simulink model "Filter2017a"  (R2017a)
settings: Solver=VariableStepAuto  StartTime=0.0  StopTime=10  RelTol=1e-3
values from neighbouring files (symbols this model uses):
  Fs = 44100    [Harjoitustyo.m]
  Hr_band = zeros(size(k))    [Harjoitustyo.m]
  Hr_high = ones(size(k))    [Harjoitustyo.m]
  Hr_low = zeros(size(k))    [Harjoitustyo.m]
  M = 64    [BuildFilter_a.m]    (also in Harjoitustyo.m; LuentoEsimerkki.m = 32)
libraries: dspsrcs4 x2
settings Model: Creator=j8889  LastModifiedBy=j8889

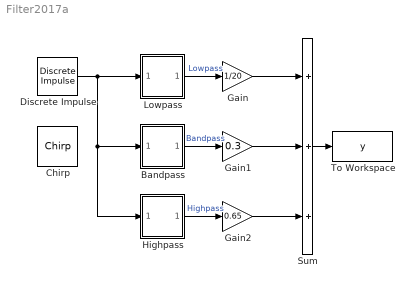
== system Filter2017a ==
  Bandpass : Subsystem
  Chirp : dspsrcs4/Chirp  sweep=Linear  mode=Unidirectional  f0=10  f1=20000  t1=10  Tsweep=50  phase=0  Ts=1/Fs  spf=1  datatype=Double  OutputFrames=off
      settings: SourceProductName=DSP System Toolbox
  Discrete Impulse : dspsrcs4/Discrete  Impulse  Delay=0  SampleTime=1  FrameSample=1  OutputFrames=off  dataType=double  isSigned=on  wordLen=16  udDataType=sfix(16)  fracBitsMode=Best precision  numFracBits=15  OutDataTypeStr=double  LastOutDataTypeStr=double
  Gain : Gain  Gain=1/20
  Gain1 : Gain  Gain=0.3
  Gain2 : Gain  Gain=0.65
  Highpass : Subsystem
  Lowpass : Subsystem
  Sum : Sum  Inputs=+++
  To Workspace : ToWorkspace  VariableName=y  SaveFormat=Timeseries  SampleTime=-1
  wires:
  Sum/1 -> To Workspace/1
  Lowpass/1(Out1) -> Gain/1  "Lowpass"
  Bandpass/1(Out1) -> Gain1/1  "Bandpass"
  Highpass/1(Out1) -> Gain2/1  "Highpass"
  Gain/1 -> Sum/1
  Gain1/1 -> Sum/2
  Gain2/1 -> Sum/3
  Discrete Impulse/1 -> Lowpass/1(In1), Highpass/1(In1), Bandpass/1(In1)

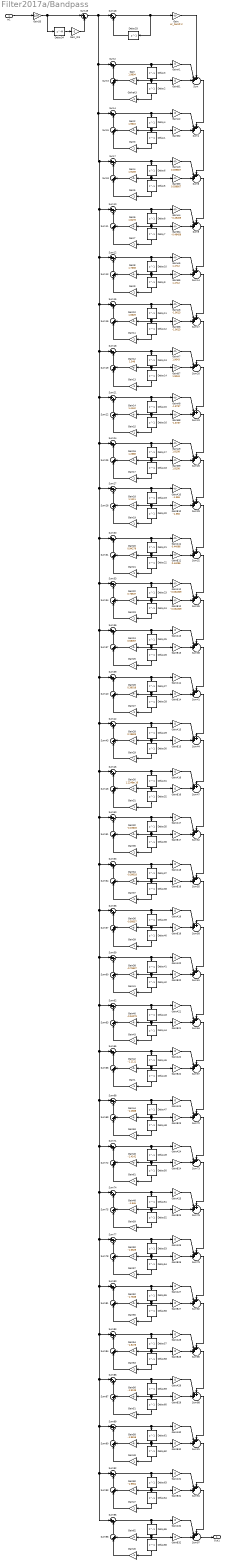
== system Filter2017a/Bandpass ==
  In1 : Inport
  Delay{1..33,35..66} (65 alike) : Delay  DelayLength=1
  Delay34 : Delay  DelayLength=M
  Gaikek3 : Gain  Gain=-1
  Gain : Gain  Gain=1.9904
  Gain{1,3,5,7,9,11,13,15,17,19,21,23,25,27,29,31,35,37,39,41,43,45,47,49,51,53,55,57,59,61,63} (31 alike) : Gain  Gain=-1
  Gain10 : Gain  Gain=1.6629
  Gain12 : Gain  Gain=1.546
  Gain14 : Gain  Gain=1.4142
  Gain16 : Gain  Gain=1.2688
  Gain18 : Gain  Gain=1.1111
  Gain2 : Gain  Gain=1.9616
  Gain20 : Gain  Gain=0.94279
  Gain22 : Gain  Gain=0.76537
  Gain24 : Gain  Gain=0.58057
  Gain26 : Gain  Gain=0.39018
  Gain28 : Gain  Gain=0.19603
  Gain30 : Gain  Gain=1.2246e-16
  Gain32 : Gain  Gain=-0.19603
  Gain33 : Gain  Gain=1/M
  Gain34 : Gain  Gain=-0.39018
  Gain36 : Gain  Gain=-0.58057
  Gain38 : Gain  Gain=-0.76537
  Gain4 : Gain  Gain=1.9139
  Gain40 : Gain  Gain=-0.94279
  Gain42 : Gain  Gain=-1.1111
  Gain44 : Gain  Gain=-1.2688
  Gain46 : Gain  Gain=-1.4142
  Gain48 : Gain  Gain=-1.546
  Gain50 : Gain  Gain=-1.6629
  Gain52 : Gain  Gain=-1.7638
  Gain54 : Gain  Gain=-1.8478
  Gain56 : Gain  Gain=-1.9139
  Gain58 : Gain  Gain=-1.9616
  Gain6 : Gain  Gain=1.8478
  Gain60 : Gain  Gain=-1.9904
  Gain62 : Gain  Gain=-2
  Gain8 : Gain  Gain=1.7638
  GainA{1..2,13..32} (22 alike) : Gain  Gain=0
  GainA10 : Gain  Gain=-1.356
  GainA11 : Gain  Gain=0.44096
  GainA12 : Gain  Gain=-0.034309
  GainA3 : Gain  Gain=0.039807
  GainA4 : Gain  Gain=-0.49459
  GainA5 : Gain  Gain=1.4712
  GainA6 : Gain  Gain=-1.9013
  GainA7 : Gain  Gain=1.9043
  GainA8 : Gain  Gain=-1.8737
  GainA9 : Gain  Gain=1.8108
  GainB{1..2,13..32} (22 alike) : Gain  Gain=0
  GainB10 : Gain  Gain=-1.356
  GainB11 : Gain  Gain=0.44096
  GainB12 : Gain  Gain=-0.034309
  GainB3 : Gain  Gain=0.039807
  GainB4 : Gain  Gain=-0.49459
  GainB5 : Gain  Gain=1.4712
  GainB6 : Gain  Gain=-1.9013
  GainB7 : Gain  Gain=1.9043
  GainB8 : Gain  Gain=-1.8737
  GainB9 : Gain  Gain=1.8108
  Gain_ : Gain  Gain=Hr_band(1)
  Gain_OG : Gain  Gain=-1
  Sum{,1,6,9,14,17,20,23,26,29,32,35,38,41,44,47,52,55,58,61,64,67,70,73,76,79,82,85,88,91,94,97} (32 alike) : Sum  Inputs=+++||
  Sum{2..5,7..8,10..13,15..16,18..19,21..22,24..25,27..28,30..31,33..34,36..37,39..40,42..43,45..46,48..51,53..54,56..57,59..60,62..63,65..66,68..69,71..72,74..75,77..78,80..81,83..84,86..87,89..90,92..93,95..96} (66 alike) : Sum  Inputs=|++
  Out1 : Outport
  wires:
  Sum47/1 -> Sum52/1
  Gain37/1 -> Sum54/1
  Gain34/1 -> Sum54/2
  Sum63/1 -> Sum62/2
  Sum58/1 -> Sum61/1
  GainA21/1 -> Sum64/2
  Delay38/1 -> Gain37/1
  Gain43/1 -> Sum63/1
  Sum54/1 -> Sum53/2
  Delay37/1 -> Delay38/1, Gain34/1, GainB18/1
  GainA18/1 -> Sum55/2
  GainB21/1 -> Sum64/3
  Sum52/1 -> Sum55/1
  Delay50/1 -> Gain61/1
  Gain32/1 -> Sum51/2
  Delay64/1 -> Gain47/1
  Delay54/1 -> Gain57/1
  Delay52/1 -> Gain59/1
  GainA19/1 -> Sum58/2
  Gain_OG/1 -> Sum49/2
  Delay62/1 -> Gain49/1
  Delay58/1 -> Gain53/1
  Sum76/1 -> Sum79/1
  Gain54/1 -> Sum84/2
  GainB24/1 -> Sum73/3
  Sum75/1 -> Sum74/2
  Sum78/1 -> Sum77/2
  Sum72/1 -> Sum71/2
  Sum80/1 -> Delay55/1, GainA27/1
  Gain57/1 -> Sum78/1
  GainA27/1 -> Sum82/2
  Gain52/1 -> Sum81/2
  Sum91/1 -> Sum94/1
  Delay55/1 -> Delay56/1, Gain52/1, GainB27/1
  Sum84/1 -> Sum83/2
  Sum93/1 -> Sum92/2
  Sum71/1 -> GainA24/1, Delay49/1
  Sum66/1 -> Sum65/2
  GainB28/1 -> Sum85/3
  Sum69/1 -> Sum68/2
  Sum92/1 -> Delay63/1, GainA31/1
  GainB25/1 -> Sum76/3
  Delay47/1 -> Delay48/1, Gain44/1, GainB23/1
  Gain49/1 -> Sum90/1
  GainA28/1 -> Sum85/2
  Sum77/1 -> GainA26/1, Delay53/1
  Delay61/1 -> GainB30/1, Gain58/1, Delay62/1
  Gain58/1 -> Sum90/2
  Delay45/1 -> GainB22/1, Gain42/1, Delay46/1
  Sum83/1 -> GainA28/1, Delay57/1
  GainA24/1 -> Sum73/2
  Gain42/1 -> Sum66/2
  Gain48/1 -> Sum75/2
  Delay66/1 -> Gain45/1
  Sum97/1 -> Out1/1
  Delay60/1 -> Gain51/1
  GainB17/1 -> Sum52/3
  Sum70/1 -> Sum73/1
  Gain39/1 -> Sum57/1
  Gain60/1 -> Sum93/2
  Sum59/1 -> Delay41/1, GainA20/1
  Delay41/1 -> Delay42/1, Gain38/1, GainB20/1
  Gain38/1 -> Sum60/2
  GainB26/1 -> Sum79/3
  Delay36/1 -> Gain35/1
  Gain35/1 -> Sum51/1
  Sum50/1 -> GainA17/1, Delay35/1
  Sum60/1 -> Sum59/2
  Sum65/1 -> GainA22/1, Delay45/1
  GainA22/1 -> Sum67/2
  GainA20/1 -> Sum61/2
  Gain41/1 -> Sum60/1
  Sum81/1 -> Sum80/2
  Sum55/1 -> Sum58/1
  Sum68/1 -> Delay47/1, GainA23/1
  Sum57/1 -> Sum56/2
  Gain36/1 -> Sum57/2
  Delay42/1 -> Gain41/1
  Gain1/1 -> Sum66/1
  GainB31/1 -> Sum94/3
  Sum64/1 -> Sum67/1
  GainB16/1 -> Sum47/3
  Delay63/1 -> Delay64/1, Gain60/1, GainB31/1
  Gain30/1 -> Sum46/2
  Sum/1 -> Sum1/1
  GainA31/1 -> Sum94/2
  Gain18/1 -> Sum28/2
  Gain25/1 -> Sum37/1
  Sum35/1 -> Sum38/1
  Sum94/1 -> Sum97/1
  Gain23/1 -> Sum34/1
  Delay32/1 -> Gain31/1
  Sum25/1 -> Sum24/2
  Gain44/1 -> Sum69/2
  Gain27/1 -> Sum40/1
  Delay13/1 -> GainB7/1, Gain12/1, Delay14/1
  GainB23/1 -> Sum70/3
  GainB5/1 -> Sum14/3
  GainA2/1 -> Sum1/2
  Gain6/1 -> Sum11/2
  Gain13/1 -> Sum19/1
  Delay27/1 -> Delay28/1, Gain26/1, GainB14/1
  Sum16/1 -> Sum15/2
  Gain55/1 -> Sum81/1
  Delay19/1 -> Delay20/1, Gain18/1, GainB10/1
  Delay25/1 -> GainB13/1, Gain24/1, Delay26/1
  Delay39/1 -> GainB19/1, Gain36/1, Delay40/1
  GainB7/1 -> Sum20/3
  Sum46/1 -> Sum45/2
  Delay16/1 -> Gain15/1
  GainA9/1 -> Sum26/2
  Sum36/1 -> GainA13/1, Delay25/1
  Sum73/1 -> Sum76/1
  Delay7/1 -> Gain7/1
  Sum6/1 -> Sum9/1
  Gain7/1 -> Sum11/1
  Delay29/1 -> GainB15/1, Gain28/1, Delay30/1
  Sum49/1 -> Sum4/1, Sum50/1, Sum53/1, Sum56/1, Sum59/1, Sum68/1, Sum71/1, Sum74/1, Sum77/1, Sum80/1, Sum83/1, Sum95/1, Sum92/1, Sum89/1, Sum86/1, Sum65/1, Sum62/1, Sum45/1, Sum42/1, Sum39/1, Sum36/1, Sum33/1, Sum30/1, Sum27/1, Sum24/1, Sum21/1, Sum18/1, Sum15/1, Sum12/1, Sum10/1, Sum7/1, Sum2/1, Sum48/1
  GainA3/1 -> Sum6/2
  Sum7/1 -> GainA3/1, Delay6/1
  Delay3/1 -> GainB1/1, Gain/1, Delay2/1
  GainB22/1 -> Sum67/3
  Delay1/1 -> Gain3/1
  GainB3/1 -> Sum6/3
  Sum33/1 -> Delay23/1, GainA12/1
  Gaikek3/1 -> Sum3/1
  Sum3/1 -> Sum2/2
  Sum11/1 -> Sum10/2
  Gain12/1 -> Sum19/2
  Gain26/1 -> Sum40/2
  Delay35/1 -> GainB17/1, Gain32/1, Delay36/1
  Sum48/1 -> Gain_/1, Delay33/1
  Gain22/1 -> Sum34/2
  Gain10/1 -> Sum16/2
  Sum43/1 -> Sum42/2
  Delay57/1 -> GainB28/1, Gain54/1, Delay58/1
  Delay6/1 -> GainB3/1, Gain4/1, Delay5/1
  Delay2/1 -> Gaikek3/1
  Delay51/1 -> Delay52/1, Gain48/1, GainB25/1
  Gain11/1 -> Sum16/1
  GainB27/1 -> Sum82/3
  Sum4/1 -> Delay4/1, GainA2/1
  Gain47/1 -> Sum93/1
  Sum53/1 -> Delay37/1, GainA18/1
  Sum13/1 -> Sum12/2
  Gain50/1 -> Sum78/2
  GainA1/1 -> Sum/2
  Gain51/1 -> Sum87/1
  GainB30/1 -> Sum91/3
  Gain31/1 -> Sum46/1
  Delay22/1 -> Gain21/1
  Gain20/1 -> Sum31/2
  Gain63/1 -> Sum69/1
  GainB13/1 -> Sum38/3
  GainA26/1 -> Sum79/2
  GainB20/1 -> Sum61/3
  Sum10/1 -> Delay8/1, GainA4/1
  Gain45/1 -> Sum96/1
  Delay30/1 -> Gain29/1
  Sum34/1 -> Sum33/2
  Sum88/1 -> Sum91/1
  Delay48/1 -> Gain63/1
  Sum19/1 -> Sum18/2
  Gain5/1 -> Sum8/1
  GainB18/1 -> Sum55/3
  Delay40/1 -> Gain39/1
  Sum90/1 -> Sum89/2
  Sum89/1 -> GainA30/1, Delay61/1
  Gain19/1 -> Sum28/1
  GainA6/1 -> Sum17/2
  Sum20/1 -> Sum23/1
  Sum39/1 -> Delay27/1, GainA14/1
  GainB14/1 -> Sum41/3
  GainA25/1 -> Sum76/2
  Sum74/1 -> Delay51/1, GainA25/1
  Sum18/1 -> GainA7/1, Delay13/1
  GainA8/1 -> Sum23/2
  Sum29/1 -> Sum32/1
  Sum1/1 -> Sum6/1
  Sum5/1 -> Sum4/2
  Delay26/1 -> Gain25/1
  Gain46/1 -> Sum72/2
  Sum12/1 -> GainA5/1, Delay10/1
  Gain61/1 -> Sum72/1
  Gain8/1 -> Sum13/2
  Delay33/1 -> Sum48/2
  Sum38/1 -> Sum41/1
  GainB4/1 -> Sum9/3
  Sum24/1 -> GainA9/1, Delay17/1
  GainA5/1 -> Sum14/2
  Delay14/1 -> Gain13/1
  GainB6/1 -> Sum17/3
  Gain14/1 -> Sum22/2
  Sum22/1 -> Sum21/2
  Delay20/1 -> Gain19/1
  GainB2/1 -> Sum1/3
  Delay8/1 -> Delay7/1, Gain6/1, GainB4/1
  Sum56/1 -> GainA19/1, Delay39/1
  GainA12/1 -> Sum35/2
  Sum82/1 -> Sum85/1
  GainA14/1 -> Sum41/2
  Delay34/1 -> Gain_OG/1
  Delay17/1 -> GainB9/1, Gain16/1, Delay18/1
  Sum23/1 -> Sum26/1
  Gain/1 -> Sum3/2
  GainA30/1 -> Sum91/2
  Delay24/1 -> Gain23/1
  GainA4/1 -> Sum9/2
  GainA16/1 -> Sum47/2
  GainB9/1 -> Sum26/3
  Sum9/1 -> Sum14/1
  Gain17/1 -> Sum25/1
  Delay44/1 -> Gain43/1
  In1/1 -> Gain33/1
  GainA23/1 -> Sum70/2
  Sum21/1 -> Delay15/1, GainA8/1
  Delay28/1 -> Gain27/1
  Gain24/1 -> Sum37/2
  Sum15/1 -> Delay11/1, GainA6/1
  GainB12/1 -> Sum35/3
  GainB10/1 -> Sum29/3
  Sum14/1 -> Sum17/1
  Delay4/1 -> Delay1/1, Gain2/1, GainB2/1
  GainA10/1 -> Sum29/2
  Delay43/1 -> GainB21/1, Gain40/1, Delay44/1
  GainB11/1 -> Sum32/3
  GainA13/1 -> Sum38/2
  GainB15/1 -> Sum44/3
  Gain59/1 -> Sum75/1
  Sum79/1 -> Sum82/1
  Delay10/1 -> GainB5/1, Gain8/1, Delay9/1
  Sum37/1 -> Sum36/2
  Sum40/1 -> Sum39/2
  Delay11/1 -> Delay12/1, Gain10/1, GainB6/1
  Sum30/1 -> GainA11/1, Delay21/1
  Sum17/1 -> Sum20/1
  Delay31/1 -> Delay32/1, Gain30/1, GainB16/1
  Delay15/1 -> Delay16/1, Gain14/1, GainB8/1
  Gain40/1 -> Sum63/2
  Sum42/1 -> GainA15/1, Delay29/1
  Gain2/1 -> Sum5/2
  Sum51/1 -> Sum50/2
  Gain15/1 -> Sum22/1
  Delay56/1 -> Gain55/1
  GainA7/1 -> Sum20/2
  Sum44/1 -> Sum47/1
  Sum8/1 -> Sum7/2
  Delay23/1 -> Delay24/1, Gain22/1, GainB12/1
  Gain16/1 -> Sum25/2
  Sum45/1 -> Delay31/1, GainA16/1
  Delay21/1 -> GainB11/1, Gain20/1, Delay22/1
  GainB1/1 -> Sum/3
  Delay18/1 -> Gain17/1
  Gain29/1 -> Sum43/1
  Gain4/1 -> Sum8/2
  Gain21/1 -> Sum31/1
  Sum27/1 -> Delay19/1, GainA10/1
  Gain28/1 -> Sum43/2
  Sum28/1 -> Sum27/2
  Delay5/1 -> Gain5/1
  Sum61/1 -> Sum64/1
  Gain56/1 -> Sum87/2
  GainB19/1 -> Sum58/3
  Sum85/1 -> Sum88/1
  Gain53/1 -> Sum84/1
  Sum41/1 -> Sum44/1
  Gain9/1 -> Sum13/1
  Delay59/1 -> Delay60/1, Gain56/1, GainB29/1
  GainA11/1 -> Sum32/2
  Sum2/1 -> GainA1/1, Delay3/1
  Sum67/1 -> Sum70/1
  GainB29/1 -> Sum88/3
  Sum87/1 -> Sum86/2
  Gain3/1 -> Sum5/1
  Sum96/1 -> Sum95/2
  Delay53/1 -> GainB26/1, Gain50/1, Delay54/1
  GainA29/1 -> Sum88/2
  GainA15/1 -> Sum44/2
  Sum26/1 -> Sum29/1
  Sum31/1 -> Sum30/2
  Delay12/1 -> Gain11/1
  Sum86/1 -> Delay59/1, GainA29/1
  Delay9/1 -> Gain9/1
  Gain33/1 -> Delay34/1, Sum49/1
  Delay46/1 -> Gain1/1
  GainB32/1 -> Sum97/3
  Sum32/1 -> Sum35/1
  Delay49/1 -> GainB24/1, Gain46/1, Delay50/1
  Sum62/1 -> GainA21/1, Delay43/1
  GainB8/1 -> Sum23/3
  Delay65/1 -> GainB32/1, Gain62/1, Delay66/1
  Gain62/1 -> Sum96/2
  Sum95/1 -> GainA32/1, Delay65/1
  GainA32/1 -> Sum97/2
  GainA17/1 -> Sum52/2
  Gain_/1 -> Sum/1

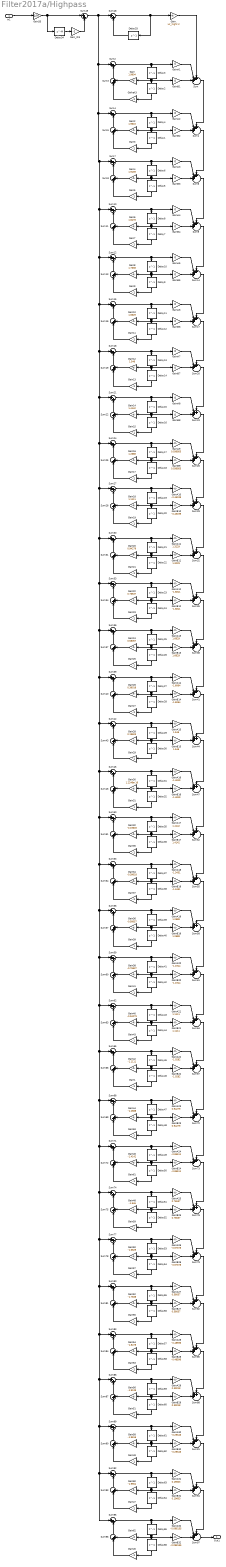
== system Filter2017a/Highpass ==
  In1 : Inport
  Delay{1..33,35..66} (65 alike) : Delay  DelayLength=1
  Delay34 : Delay  DelayLength=M
  Gaikek3 : Gain  Gain=-1
  Gain : Gain  Gain=1.9904
  Gain{1,3,5,7,9,11,13,15,17,19,21,23,25,27,29,31,35,37,39,41,43,45,47,49,51,53,55,57,59,61,63} (31 alike) : Gain  Gain=-1
  Gain10 : Gain  Gain=1.6629
  Gain12 : Gain  Gain=1.546
  Gain14 : Gain  Gain=1.4142
  Gain16 : Gain  Gain=1.2688
  Gain18 : Gain  Gain=1.1111
  Gain2 : Gain  Gain=1.9616
  Gain20 : Gain  Gain=0.94279
  Gain22 : Gain  Gain=0.76537
  Gain24 : Gain  Gain=0.58057
  Gain26 : Gain  Gain=0.39018
  Gain28 : Gain  Gain=0.19603
  Gain30 : Gain  Gain=1.2246e-16
  Gain32 : Gain  Gain=-0.19603
  Gain33 : Gain  Gain=1/M
  Gain34 : Gain  Gain=-0.39018
  Gain36 : Gain  Gain=-0.58057
  Gain38 : Gain  Gain=-0.76537
  Gain4 : Gain  Gain=1.9139
  Gain40 : Gain  Gain=-0.94279
  Gain42 : Gain  Gain=-1.1111
  Gain44 : Gain  Gain=-1.2688
  Gain46 : Gain  Gain=-1.4142
  Gain48 : Gain  Gain=-1.546
  Gain50 : Gain  Gain=-1.6629
  Gain52 : Gain  Gain=-1.7638
  Gain54 : Gain  Gain=-1.8478
  Gain56 : Gain  Gain=-1.9139
  Gain58 : Gain  Gain=-1.9616
  Gain6 : Gain  Gain=1.8478
  Gain60 : Gain  Gain=-1.9904
  Gain62 : Gain  Gain=-2
  Gain8 : Gain  Gain=1.7638
  GainA{1..8} (8 alike) : Gain  Gain=0
  GainA10 : Gain  Gain=-0.45199
  GainA11 : Gain  Gain=1.3229
  GainA12 : Gain  Gain=-1.6811
  GainA13 : Gain  Gain=1.6629
  GainA14 : Gain  Gain=-1.6064
  GainA15 : Gain  Gain=1.546
  GainA16 : Gain  Gain=-1.4819
  GainA17 : Gain  Gain=1.4142
  GainA18 : Gain  Gain=-1.3431
  GainA19 : Gain  Gain=1.2688
  GainA20 : Gain  Gain=-1.1914
  GainA21 : Gain  Gain=1.1111
  GainA22 : Gain  Gain=-1.0282
  GainA23 : Gain  Gain=0.94279
  GainA24 : Gain  Gain=-0.85511
  GainA25 : Gain  Gain=0.76537
  GainA26 : Gain  Gain=-0.67378
  GainA27 : Gain  Gain=0.58057
  GainA28 : Gain  Gain=-0.48596
  GainA29 : Gain  Gain=0.39018
  GainA30 : Gain  Gain=-0.29346
  GainA31 : Gain  Gain=0.19603
  GainA32 : Gain  Gain=-0.098135
  GainA9 : Gain  Gain=0.036955
  GainB{1..8} (8 alike) : Gain  Gain=0
  GainB10 : Gain  Gain=-0.45199
  GainB11 : Gain  Gain=1.3229
  GainB12 : Gain  Gain=-1.6811
  GainB13 : Gain  Gain=1.6629
  GainB14 : Gain  Gain=-1.6064
  GainB15 : Gain  Gain=1.546
  GainB16 : Gain  Gain=-1.4819
  GainB17 : Gain  Gain=1.4142
  GainB18 : Gain  Gain=-1.3431
  GainB19 : Gain  Gain=1.2688
  GainB20 : Gain  Gain=-1.1914
  GainB21 : Gain  Gain=1.1111
  GainB22 : Gain  Gain=-1.0282
  GainB23 : Gain  Gain=0.94279
  GainB24 : Gain  Gain=-0.85511
  GainB25 : Gain  Gain=0.76537
  GainB26 : Gain  Gain=-0.67378
  GainB27 : Gain  Gain=0.58057
  GainB28 : Gain  Gain=-0.48596
  GainB29 : Gain  Gain=0.39018
  GainB30 : Gain  Gain=-0.29346
  GainB31 : Gain  Gain=0.19603
  GainB32 : Gain  Gain=-0.098135
  GainB9 : Gain  Gain=0.036955
  Gain_ : Gain  Gain=Hr_high(1)
  Gain_OG : Gain  Gain=-1
  Sum{,1,6,9,14,17,20,23,26,29,32,35,38,41,44,47,52,55,58,61,64,67,70,73,76,79,82,85,88,91,94,97} (32 alike) : Sum  Inputs=+++||
  Sum{2..5,7..8,10..13,15..16,18..19,21..22,24..25,27..28,30..31,33..34,36..37,39..40,42..43,45..46,48..51,53..54,56..57,59..60,62..63,65..66,68..69,71..72,74..75,77..78,80..81,83..84,86..87,89..90,92..93,95..96} (66 alike) : Sum  Inputs=|++
  Out1 : Outport
  wires:
  Sum47/1 -> Sum52/1
  Gain37/1 -> Sum54/1
  Gain34/1 -> Sum54/2
  Sum63/1 -> Sum62/2
  Sum58/1 -> Sum61/1
  GainA21/1 -> Sum64/2
  Delay38/1 -> Gain37/1
  Gain43/1 -> Sum63/1
  Sum54/1 -> Sum53/2
  Delay37/1 -> Delay38/1, Gain34/1, GainB18/1
  GainA18/1 -> Sum55/2
  GainB21/1 -> Sum64/3
  Sum52/1 -> Sum55/1
  Delay50/1 -> Gain61/1
  Gain32/1 -> Sum51/2
  Delay64/1 -> Gain47/1
  Delay54/1 -> Gain57/1
  Delay52/1 -> Gain59/1
  GainA19/1 -> Sum58/2
  Gain_OG/1 -> Sum49/2
  Delay62/1 -> Gain49/1
  Delay58/1 -> Gain53/1
  Sum76/1 -> Sum79/1
  Gain54/1 -> Sum84/2
  GainB24/1 -> Sum73/3
  Sum75/1 -> Sum74/2
  Sum78/1 -> Sum77/2
  Sum72/1 -> Sum71/2
  Sum80/1 -> Delay55/1, GainA27/1
  Gain57/1 -> Sum78/1
  GainA27/1 -> Sum82/2
  Gain52/1 -> Sum81/2
  Sum91/1 -> Sum94/1
  Delay55/1 -> Delay56/1, Gain52/1, GainB27/1
  Sum84/1 -> Sum83/2
  Sum93/1 -> Sum92/2
  Sum71/1 -> GainA24/1, Delay49/1
  Sum66/1 -> Sum65/2
  GainB28/1 -> Sum85/3
  Sum69/1 -> Sum68/2
  Sum92/1 -> Delay63/1, GainA31/1
  GainB25/1 -> Sum76/3
  Delay47/1 -> Delay48/1, Gain44/1, GainB23/1
  Gain49/1 -> Sum90/1
  GainA28/1 -> Sum85/2
  Sum77/1 -> GainA26/1, Delay53/1
  Delay61/1 -> GainB30/1, Gain58/1, Delay62/1
  Gain58/1 -> Sum90/2
  Delay45/1 -> GainB22/1, Gain42/1, Delay46/1
  Sum83/1 -> GainA28/1, Delay57/1
  GainA24/1 -> Sum73/2
  Gain42/1 -> Sum66/2
  Gain48/1 -> Sum75/2
  Delay66/1 -> Gain45/1
  Sum97/1 -> Out1/1
  Delay60/1 -> Gain51/1
  GainB17/1 -> Sum52/3
  Sum70/1 -> Sum73/1
  Gain39/1 -> Sum57/1
  Gain60/1 -> Sum93/2
  Sum59/1 -> Delay41/1, GainA20/1
  Delay41/1 -> Delay42/1, Gain38/1, GainB20/1
  Gain38/1 -> Sum60/2
  GainB26/1 -> Sum79/3
  Delay36/1 -> Gain35/1
  Gain35/1 -> Sum51/1
  Sum50/1 -> GainA17/1, Delay35/1
  Sum60/1 -> Sum59/2
  Sum65/1 -> GainA22/1, Delay45/1
  GainA22/1 -> Sum67/2
  GainA20/1 -> Sum61/2
  Gain41/1 -> Sum60/1
  Sum81/1 -> Sum80/2
  Sum55/1 -> Sum58/1
  Sum68/1 -> Delay47/1, GainA23/1
  Sum57/1 -> Sum56/2
  Gain36/1 -> Sum57/2
  Delay42/1 -> Gain41/1
  Gain1/1 -> Sum66/1
  GainB31/1 -> Sum94/3
  Sum64/1 -> Sum67/1
  GainB16/1 -> Sum47/3
  Delay63/1 -> Delay64/1, Gain60/1, GainB31/1
  Gain30/1 -> Sum46/2
  Sum/1 -> Sum1/1
  GainA31/1 -> Sum94/2
  Gain18/1 -> Sum28/2
  Gain25/1 -> Sum37/1
  Sum35/1 -> Sum38/1
  Sum94/1 -> Sum97/1
  Gain23/1 -> Sum34/1
  Delay32/1 -> Gain31/1
  Sum25/1 -> Sum24/2
  Gain44/1 -> Sum69/2
  Gain27/1 -> Sum40/1
  Delay13/1 -> GainB7/1, Gain12/1, Delay14/1
  GainB23/1 -> Sum70/3
  GainB5/1 -> Sum14/3
  GainA2/1 -> Sum1/2
  Gain6/1 -> Sum11/2
  Gain13/1 -> Sum19/1
  Delay27/1 -> Delay28/1, Gain26/1, GainB14/1
  Sum16/1 -> Sum15/2
  Gain55/1 -> Sum81/1
  Delay19/1 -> Delay20/1, Gain18/1, GainB10/1
  Delay25/1 -> GainB13/1, Gain24/1, Delay26/1
  Delay39/1 -> GainB19/1, Gain36/1, Delay40/1
  GainB7/1 -> Sum20/3
  Sum46/1 -> Sum45/2
  Delay16/1 -> Gain15/1
  GainA9/1 -> Sum26/2
  Sum36/1 -> GainA13/1, Delay25/1
  Sum73/1 -> Sum76/1
  Delay7/1 -> Gain7/1
  Sum6/1 -> Sum9/1
  Gain7/1 -> Sum11/1
  Delay29/1 -> GainB15/1, Gain28/1, Delay30/1
  Sum49/1 -> Sum4/1, Sum50/1, Sum53/1, Sum56/1, Sum59/1, Sum68/1, Sum71/1, Sum74/1, Sum77/1, Sum80/1, Sum83/1, Sum95/1, Sum92/1, Sum89/1, Sum86/1, Sum65/1, Sum62/1, Sum45/1, Sum42/1, Sum39/1, Sum36/1, Sum33/1, Sum30/1, Sum27/1, Sum24/1, Sum21/1, Sum18/1, Sum15/1, Sum12/1, Sum10/1, Sum7/1, Sum2/1, Sum48/1
  GainA3/1 -> Sum6/2
  Sum7/1 -> GainA3/1, Delay6/1
  Delay3/1 -> GainB1/1, Gain/1, Delay2/1
  GainB22/1 -> Sum67/3
  Delay1/1 -> Gain3/1
  GainB3/1 -> Sum6/3
  Sum33/1 -> Delay23/1, GainA12/1
  Gaikek3/1 -> Sum3/1
  Sum3/1 -> Sum2/2
  Sum11/1 -> Sum10/2
  Gain12/1 -> Sum19/2
  Gain26/1 -> Sum40/2
  Delay35/1 -> GainB17/1, Gain32/1, Delay36/1
  Sum48/1 -> Gain_/1, Delay33/1
  Gain22/1 -> Sum34/2
  Gain10/1 -> Sum16/2
  Sum43/1 -> Sum42/2
  Delay57/1 -> GainB28/1, Gain54/1, Delay58/1
  Delay6/1 -> GainB3/1, Gain4/1, Delay5/1
  Delay2/1 -> Gaikek3/1
  Delay51/1 -> Delay52/1, Gain48/1, GainB25/1
  Gain11/1 -> Sum16/1
  GainB27/1 -> Sum82/3
  Sum4/1 -> Delay4/1, GainA2/1
  Gain47/1 -> Sum93/1
  Sum53/1 -> Delay37/1, GainA18/1
  Sum13/1 -> Sum12/2
  Gain50/1 -> Sum78/2
  GainA1/1 -> Sum/2
  Gain51/1 -> Sum87/1
  GainB30/1 -> Sum91/3
  Gain31/1 -> Sum46/1
  Delay22/1 -> Gain21/1
  Gain20/1 -> Sum31/2
  Gain63/1 -> Sum69/1
  GainB13/1 -> Sum38/3
  GainA26/1 -> Sum79/2
  GainB20/1 -> Sum61/3
  Sum10/1 -> Delay8/1, GainA4/1
  Gain45/1 -> Sum96/1
  Delay30/1 -> Gain29/1
  Sum34/1 -> Sum33/2
  Sum88/1 -> Sum91/1
  Delay48/1 -> Gain63/1
  Sum19/1 -> Sum18/2
  Gain5/1 -> Sum8/1
  GainB18/1 -> Sum55/3
  Delay40/1 -> Gain39/1
  Sum90/1 -> Sum89/2
  Sum89/1 -> GainA30/1, Delay61/1
  Gain19/1 -> Sum28/1
  GainA6/1 -> Sum17/2
  Sum20/1 -> Sum23/1
  Sum39/1 -> Delay27/1, GainA14/1
  GainB14/1 -> Sum41/3
  GainA25/1 -> Sum76/2
  Sum74/1 -> Delay51/1, GainA25/1
  Sum18/1 -> GainA7/1, Delay13/1
  GainA8/1 -> Sum23/2
  Sum29/1 -> Sum32/1
  Sum1/1 -> Sum6/1
  Sum5/1 -> Sum4/2
  Delay26/1 -> Gain25/1
  Gain46/1 -> Sum72/2
  Sum12/1 -> GainA5/1, Delay10/1
  Gain61/1 -> Sum72/1
  Gain8/1 -> Sum13/2
  Delay33/1 -> Sum48/2
  Sum38/1 -> Sum41/1
  GainB4/1 -> Sum9/3
  Sum24/1 -> GainA9/1, Delay17/1
  GainA5/1 -> Sum14/2
  Delay14/1 -> Gain13/1
  GainB6/1 -> Sum17/3
  Gain14/1 -> Sum22/2
  Sum22/1 -> Sum21/2
  Delay20/1 -> Gain19/1
  GainB2/1 -> Sum1/3
  Delay8/1 -> Delay7/1, Gain6/1, GainB4/1
  Sum56/1 -> GainA19/1, Delay39/1
  GainA12/1 -> Sum35/2
  Sum82/1 -> Sum85/1
  GainA14/1 -> Sum41/2
  Delay34/1 -> Gain_OG/1
  Delay17/1 -> GainB9/1, Gain16/1, Delay18/1
  Sum23/1 -> Sum26/1
  Gain/1 -> Sum3/2
  GainA30/1 -> Sum91/2
  Delay24/1 -> Gain23/1
  GainA4/1 -> Sum9/2
  GainA16/1 -> Sum47/2
  GainB9/1 -> Sum26/3
  Sum9/1 -> Sum14/1
  Gain17/1 -> Sum25/1
  Delay44/1 -> Gain43/1
  In1/1 -> Gain33/1
  GainA23/1 -> Sum70/2
  Sum21/1 -> Delay15/1, GainA8/1
  Delay28/1 -> Gain27/1
  Gain24/1 -> Sum37/2
  Sum15/1 -> Delay11/1, GainA6/1
  GainB12/1 -> Sum35/3
  GainB10/1 -> Sum29/3
  Sum14/1 -> Sum17/1
  Delay4/1 -> Delay1/1, Gain2/1, GainB2/1
  GainA10/1 -> Sum29/2
  Delay43/1 -> GainB21/1, Gain40/1, Delay44/1
  GainB11/1 -> Sum32/3
  GainA13/1 -> Sum38/2
  GainB15/1 -> Sum44/3
  Gain59/1 -> Sum75/1
  Sum79/1 -> Sum82/1
  Delay10/1 -> GainB5/1, Gain8/1, Delay9/1
  Sum37/1 -> Sum36/2
  Sum40/1 -> Sum39/2
  Delay11/1 -> Delay12/1, Gain10/1, GainB6/1
  Sum30/1 -> GainA11/1, Delay21/1
  Sum17/1 -> Sum20/1
  Delay31/1 -> Delay32/1, Gain30/1, GainB16/1
  Delay15/1 -> Delay16/1, Gain14/1, GainB8/1
  Gain40/1 -> Sum63/2
  Sum42/1 -> GainA15/1, Delay29/1
  Gain2/1 -> Sum5/2
  Sum51/1 -> Sum50/2
  Gain15/1 -> Sum22/1
  Delay56/1 -> Gain55/1
  GainA7/1 -> Sum20/2
  Sum44/1 -> Sum47/1
  Sum8/1 -> Sum7/2
  Delay23/1 -> Delay24/1, Gain22/1, GainB12/1
  Gain16/1 -> Sum25/2
  Sum45/1 -> Delay31/1, GainA16/1
  Delay21/1 -> GainB11/1, Gain20/1, Delay22/1
  GainB1/1 -> Sum/3
  Delay18/1 -> Gain17/1
  Gain29/1 -> Sum43/1
  Gain4/1 -> Sum8/2
  Gain21/1 -> Sum31/1
  Sum27/1 -> Delay19/1, GainA10/1
  Gain28/1 -> Sum43/2
  Sum28/1 -> Sum27/2
  Delay5/1 -> Gain5/1
  Sum61/1 -> Sum64/1
  Gain56/1 -> Sum87/2
  GainB19/1 -> Sum58/3
  Sum85/1 -> Sum88/1
  Gain53/1 -> Sum84/1
  Sum41/1 -> Sum44/1
  Gain9/1 -> Sum13/1
  Delay59/1 -> Delay60/1, Gain56/1, GainB29/1
  GainA11/1 -> Sum32/2
  Sum2/1 -> GainA1/1, Delay3/1
  Sum67/1 -> Sum70/1
  GainB29/1 -> Sum88/3
  Sum87/1 -> Sum86/2
  Gain3/1 -> Sum5/1
  Sum96/1 -> Sum95/2
  Delay53/1 -> GainB26/1, Gain50/1, Delay54/1
  GainA29/1 -> Sum88/2
  GainA15/1 -> Sum44/2
  Sum26/1 -> Sum29/1
  Sum31/1 -> Sum30/2
  Delay12/1 -> Gain11/1
  Sum86/1 -> Delay59/1, GainA29/1
  Delay9/1 -> Gain9/1
  Gain33/1 -> Delay34/1, Sum49/1
  Delay46/1 -> Gain1/1
  GainB32/1 -> Sum97/3
  Sum32/1 -> Sum35/1
  Delay49/1 -> GainB24/1, Gain46/1, Delay50/1
  Sum62/1 -> GainA21/1, Delay43/1
  GainB8/1 -> Sum23/3
  Delay65/1 -> GainB32/1, Gain62/1, Delay66/1
  Gain62/1 -> Sum96/2
  Sum95/1 -> GainA32/1, Delay65/1
  GainA32/1 -> Sum97/2
  GainA17/1 -> Sum52/2
  Gain_/1 -> Sum/1

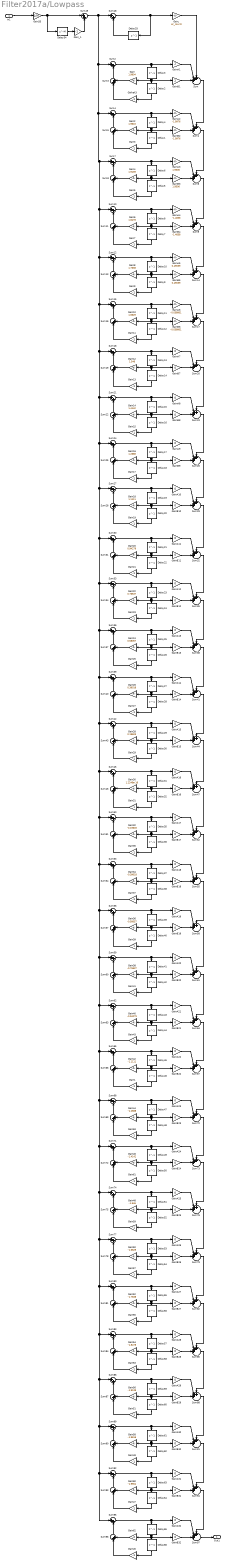
== system Filter2017a/Lowpass ==
  In1 : Inport
  Delay{1..33,35..66} (65 alike) : Delay  DelayLength=1
  Delay34 : Delay  DelayLength=M
  Gaikek3 : Gain  Gain=-1
  Gain : Gain  Gain=1.9904
  Gain{1,3,5,7,9,11,13,15,17,19,21,23,25,27,29,31,35,37,39,41,43,45,47,49,51,53,55,57,59,61,63} (31 alike) : Gain  Gain=-1
  Gain10 : Gain  Gain=1.6629
  Gain12 : Gain  Gain=1.546
  Gain14 : Gain  Gain=1.4142
  Gain16 : Gain  Gain=1.2688
  Gain18 : Gain  Gain=1.1111
  Gain2 : Gain  Gain=1.9616
  Gain20 : Gain  Gain=0.94279
  Gain22 : Gain  Gain=0.76537
  Gain24 : Gain  Gain=0.58057
  Gain26 : Gain  Gain=0.39018
  Gain28 : Gain  Gain=0.19603
  Gain30 : Gain  Gain=1.2246e-16
  Gain32 : Gain  Gain=-0.19603
  Gain33 : Gain  Gain=1/M
  Gain34 : Gain  Gain=-0.39018
  Gain36 : Gain  Gain=-0.58057
  Gain38 : Gain  Gain=-0.76537
  Gain4 : Gain  Gain=1.9139
  Gain40 : Gain  Gain=-0.94279
  Gain42 : Gain  Gain=-1.1111
  Gain44 : Gain  Gain=-1.2688
  Gain46 : Gain  Gain=-1.4142
  Gain48 : Gain  Gain=-1.546
  Gain50 : Gain  Gain=-1.6629
  Gain52 : Gain  Gain=-1.7638
  Gain54 : Gain  Gain=-1.8478
  Gain56 : Gain  Gain=-1.9139
  Gain58 : Gain  Gain=-1.9616
  Gain6 : Gain  Gain=1.8478
  Gain60 : Gain  Gain=-1.9904
  Gain62 : Gain  Gain=-2
  Gain8 : Gain  Gain=1.7638
  GainA1 : Gain  Gain=2
  GainA{7..32} (26 alike) : Gain  Gain=0
  GainA2 : Gain  Gain=-1.9976
  GainA3 : Gain  Gain=1.9506
  GainA4 : Gain  Gain=-1.4838
  GainA5 : Gain  Gain=0.49039
  GainA6 : Gain  Gain=-0.038801
  GainB1 : Gain  Gain=2
  GainB{7..32} (26 alike) : Gain  Gain=0
  GainB2 : Gain  Gain=-1.9976
  GainB3 : Gain  Gain=1.9506
  GainB4 : Gain  Gain=-1.4838
  GainB5 : Gain  Gain=0.49039
  GainB6 : Gain  Gain=-0.038801
  Gain_ : Gain  Gain=Hr_low(1)
  Gain_1 : Gain  Gain=-1
  Sum{,1,6,9,14,17,20,23,26,29,32,35,38,41,44,47,52,55,58,61,64,67,70,73,76,79,82,85,88,91,94,97} (32 alike) : Sum  Inputs=+++||
  Sum{2..5,7..8,10..13,15..16,18..19,21..22,24..25,27..28,30..31,33..34,36..37,39..40,42..43,45..46,48..51,53..54,56..57,59..60,62..63,65..66,68..69,71..72,74..75,77..78,80..81,83..84,86..87,89..90,92..93,95..96} (66 alike) : Sum  Inputs=|++
  Out1 : Outport
  wires:
  Sum97/1 -> Out1/1
  Gain46/1 -> Sum72/2
  Delay49/1 -> Delay50/1, Gain46/1, GainB24/1
  GainB24/1 -> Sum73/3
  GainA24/1 -> Sum73/2
  Sum70/1 -> Sum73/1
  Delay50/1 -> Gain61/1
  Gain61/1 -> Sum72/1
  Sum72/1 -> Sum71/2
  Sum71/1 -> Delay49/1, GainA24/1
  Gain55/1 -> Sum81/1
  Sum81/1 -> Sum80/2
  GainB27/1 -> Sum82/3
  GainA27/1 -> Sum82/2
  Sum80/1 -> GainA27/1, Delay55/1
  Gain52/1 -> Sum81/2
  Delay55/1 -> GainB27/1, Gain52/1, Delay56/1
  Delay56/1 -> Gain55/1
  Sum76/1 -> Sum79/1
  Sum82/1 -> Sum85/1
  Delay53/1 -> Delay54/1, Gain50/1, GainB26/1
  Gain50/1 -> Sum78/2
  Sum77/1 -> Delay53/1, GainA26/1
  GainA26/1 -> Sum79/2
  Sum67/1 -> Sum70/1
  Delay54/1 -> Gain57/1
  Gain57/1 -> Sum78/1
  GainB26/1 -> Sum79/3
  Sum78/1 -> Sum77/2
  Delay57/1 -> Delay58/1, Gain54/1, GainB28/1
  GainA28/1 -> Sum85/2
  GainB28/1 -> Sum85/3
  Sum83/1 -> Delay57/1, GainA28/1
  Sum84/1 -> Sum83/2
  Gain54/1 -> Sum84/2
  Sum79/1 -> Sum82/1
  Delay58/1 -> Gain53/1
  Gain53/1 -> Sum84/1
  Sum69/1 -> Sum68/2
  Sum74/1 -> GainA25/1, Delay51/1
  GainB25/1 -> Sum76/3
  Sum66/1 -> Sum65/2
  Sum65/1 -> Delay45/1, GainA22/1
  Sum68/1 -> GainA23/1, Delay47/1
  Delay46/1 -> Gain1/1
  Gain1/1 -> Sum66/1
  GainB22/1 -> Sum67/3
  Gain63/1 -> Sum69/1
  Sum64/1 -> Sum67/1
  Gain48/1 -> Sum75/2
  Delay48/1 -> Gain63/1
  GainA23/1 -> Sum70/2
  GainB23/1 -> Sum70/3
  Gain44/1 -> Sum69/2
  Gain42/1 -> Sum66/2
  Delay45/1 -> Delay46/1, Gain42/1, GainB22/1
  GainA22/1 -> Sum67/2
  GainA25/1 -> Sum76/2
  Gain59/1 -> Sum75/1
  Sum75/1 -> Sum74/2
  Delay51/1 -> GainB25/1, Gain48/1, Delay52/1
  Delay52/1 -> Gain59/1
  Delay47/1 -> GainB23/1, Gain44/1, Delay48/1
  Sum73/1 -> Sum76/1
  Sum88/1 -> Sum91/1
  Delay62/1 -> Gain49/1
  Delay61/1 -> Delay62/1, Gain58/1, GainB30/1
  Sum90/1 -> Sum89/2
  Gain49/1 -> Sum90/1
  GainA30/1 -> Sum91/2
  Gain58/1 -> Sum90/2
  GainB30/1 -> Sum91/3
  Sum89/1 -> Delay61/1, GainA30/1
  Sum94/1 -> Sum97/1
  Sum93/1 -> Sum92/2
  GainB31/1 -> Sum94/3
  Gain47/1 -> Sum93/1
  Delay64/1 -> Gain47/1
  GainA31/1 -> Sum94/2
  Sum92/1 -> GainA31/1, Delay63/1
  Gain60/1 -> Sum93/2
  Delay63/1 -> GainB31/1, Gain60/1, Delay64/1
  Sum91/1 -> Sum94/1
  Delay66/1 -> Gain45/1
  Delay65/1 -> Delay66/1, Gain62/1, GainB32/1
  Gain62/1 -> Sum96/2
  Sum95/1 -> Delay65/1, GainA32/1
  GainA32/1 -> Sum97/2
  GainB32/1 -> Sum97/3
  Sum96/1 -> Sum95/2
  Gain45/1 -> Sum96/1
  Sum86/1 -> GainA29/1, Delay59/1
  Sum87/1 -> Sum86/2
  Gain51/1 -> Sum87/1
  Delay60/1 -> Gain51/1
  Sum85/1 -> Sum88/1
  GainA29/1 -> Sum88/2
  GainB29/1 -> Sum88/3
  Delay59/1 -> GainB29/1, Gain56/1, Delay60/1
  Gain56/1 -> Sum87/2
  Sum61/1 -> Sum64/1
  Gain32/1 -> Sum51/2
  Delay35/1 -> Delay36/1, Gain32/1, GainB17/1
  GainB17/1 -> Sum52/3
  GainA17/1 -> Sum52/2
  Sum47/1 -> Sum52/1
  Delay36/1 -> Gain35/1
  Gain35/1 -> Sum51/1
  Sum51/1 -> Sum50/2
  Sum50/1 -> Delay35/1, GainA17/1
  Gain41/1 -> Sum60/1
  Sum60/1 -> Sum59/2
  GainB20/1 -> Sum61/3
  GainA20/1 -> Sum61/2
  Sum59/1 -> GainA20/1, Delay41/1
  Gain38/1 -> Sum60/2
  Delay41/1 -> GainB20/1, Gain38/1, Delay42/1
  Delay42/1 -> Gain41/1
  Sum55/1 -> Sum58/1
  Delay39/1 -> Delay40/1, Gain36/1, GainB19/1
  Gain36/1 -> Sum57/2
  Sum56/1 -> Delay39/1, GainA19/1
  GainA19/1 -> Sum58/2
  Delay40/1 -> Gain39/1
  Gain39/1 -> Sum57/1
  GainB19/1 -> Sum58/3
  Sum57/1 -> Sum56/2
  Delay43/1 -> Delay44/1, Gain40/1, GainB21/1
  GainA21/1 -> Sum64/2
  GainB21/1 -> Sum64/3
  Sum62/1 -> Delay43/1, GainA21/1
  Sum63/1 -> Sum62/2
  Gain40/1 -> Sum63/2
  Sum58/1 -> Sum61/1
  Delay44/1 -> Gain43/1
  Gain43/1 -> Sum63/1
  Sum53/1 -> GainA18/1, Delay37/1
  GainB18/1 -> Sum55/3
  Gain34/1 -> Sum54/2
  GainA18/1 -> Sum55/2
  Gain37/1 -> Sum54/1
  Sum54/1 -> Sum53/2
  Delay37/1 -> GainB18/1, Gain34/1, Delay38/1
  Delay38/1 -> Gain37/1
  Sum52/1 -> Sum55/1
  Sum2/1 -> Delay3/1, GainA1/1
  Sum35/1 -> Sum38/1
  Sum/1 -> Sum1/1
  Delay21/1 -> Delay22/1, Gain20/1, GainB11/1
  Sum20/1 -> Sum23/1
  Delay26/1 -> Gain25/1
  Sum1/1 -> Sum6/1
  Delay25/1 -> Delay26/1, Gain24/1, GainB13/1
  Sum37/1 -> Sum36/2
  Gain25/1 -> Sum37/1
  GainA13/1 -> Sum38/2
  GainA10/1 -> Sum29/2
  Delay19/1 -> GainB10/1, Gain18/1, Delay20/1
  Gain18/1 -> Sum28/2
  Gain20/1 -> Sum31/2
  GainB11/1 -> Sum32/3
  GainA11/1 -> Sum32/2
  Delay22/1 -> Gain21/1
  Gain24/1 -> Sum37/2
  Sum26/1 -> Sum29/1
  Gain21/1 -> Sum31/1
  GainB10/1 -> Sum29/3
  Gain19/1 -> Sum28/1
  Delay20/1 -> Gain19/1
  Sum30/1 -> Delay21/1, GainA11/1
  Sum27/1 -> GainA10/1, Delay19/1
  Sum28/1 -> Sum27/2
  GainB13/1 -> Sum38/3
  Sum36/1 -> Delay25/1, GainA13/1
  Sum31/1 -> Sum30/2
  Sum14/1 -> Sum17/1
  Gain31/1 -> Sum46/1
  Delay32/1 -> Gain31/1
  Sum41/1 -> Sum44/1
  Gain33/1 -> Sum49/1, Delay34/1
  Gain30/1 -> Sum46/2
  Gain9/1 -> Sum13/1
  Delay9/1 -> Gain9/1
  Gain8/1 -> Sum13/2
  GainB5/1 -> Sum14/3
  Delay10/1 -> Delay9/1, Gain8/1, GainB5/1
  Sum13/1 -> Sum12/2
  GainA5/1 -> Sum14/2
  Sum46/1 -> Sum45/2
  Sum45/1 -> GainA16/1, Delay31/1
  GainB16/1 -> Sum47/3
  GainA16/1 -> Sum47/2
  Sum12/1 -> Delay10/1, GainA5/1
  Sum9/1 -> Sum14/1
  Delay31/1 -> GainB16/1, Gain30/1, Delay32/1
  Sum40/1 -> Sum39/2
  GainB14/1 -> Sum41/3
  Gain27/1 -> Sum40/1
  Delay28/1 -> Gain27/1
  Sum29/1 -> Sum32/1
  GainA14/1 -> Sum41/2
  Sum39/1 -> GainA14/1, Delay27/1
  Gain26/1 -> Sum40/2
  Delay27/1 -> GainB14/1, Gain26/1, Delay28/1
  Delay34/1 -> Gain_1/1
  Sum17/1 -> Sum20/1
  Sum6/1 -> Sum9/1
  Sum3/1 -> Sum2/2
  Sum8/1 -> Sum7/2
  Sum44/1 -> Sum47/1
  Gain/1 -> Sum3/2
  Gaikek3/1 -> Sum3/1
  Sum7/1 -> Delay6/1, GainA3/1
  Delay5/1 -> Gain5/1
  Gain5/1 -> Sum8/1
  Delay6/1 -> Delay5/1, Gain4/1, GainB3/1
  GainB3/1 -> Sum6/3
  GainA3/1 -> Sum6/2
  Delay3/1 -> Delay2/1, Gain/1, GainB1/1
  Delay2/1 -> Gaikek3/1
  Gain4/1 -> Sum8/2
  Sum38/1 -> Sum41/1
  Delay18/1 -> Gain17/1
  Gain16/1 -> Sum25/2
  GainB7/1 -> Sum20/3
  Delay13/1 -> Delay14/1, Gain12/1, GainB7/1
  Sum18/1 -> Delay13/1, GainA7/1
  Delay15/1 -> GainB8/1, Gain14/1, Delay16/1
  Sum21/1 -> GainA8/1, Delay15/1
  Sum24/1 -> Delay17/1, GainA9/1
  GainA7/1 -> Sum20/2
  Delay14/1 -> Gain13/1
  Delay17/1 -> Delay18/1, Gain16/1, GainB9/1
  Gain17/1 -> Sum25/1
  Delay16/1 -> Gain15/1
  GainA8/1 -> Sum23/2
  Sum19/1 -> Sum18/2
  GainB9/1 -> Sum26/3
  Gain14/1 -> Sum22/2
  Gain12/1 -> Sum19/2
  Sum22/1 -> Sum21/2
  GainB8/1 -> Sum23/3
  Gain13/1 -> Sum19/1
  GainA9/1 -> Sum26/2
  Gain15/1 -> Sum22/1
  Sum25/1 -> Sum24/2
  Delay33/1 -> Sum48/2
  Sum48/1 -> Delay33/1, Gain_/1
  Delay12/1 -> Gain11/1
  Sum15/1 -> GainA6/1, Delay11/1
  Sum16/1 -> Sum15/2
  GainB6/1 -> Sum17/3
  Gain10/1 -> Sum16/2
  Delay11/1 -> GainB6/1, Gain10/1, Delay12/1
  Gain11/1 -> Sum16/1
  GainA6/1 -> Sum17/2
  Delay30/1 -> Gain29/1
  Sum4/1 -> GainA2/1, Delay4/1
  GainB2/1 -> Sum1/3
  Delay29/1 -> Delay30/1, Gain28/1, GainB15/1
  Gain28/1 -> Sum43/2
  Sum42/1 -> Delay29/1, GainA15/1
  GainA2/1 -> Sum1/2
  GainA15/1 -> Sum44/2
  GainB15/1 -> Sum44/3
  Delay1/1 -> Gain3/1
  Gain2/1 -> Sum5/2
  Sum43/1 -> Sum42/2
  Delay4/1 -> GainB2/1, Gain2/1, Delay1/1
  Sum5/1 -> Sum4/2
  Gain29/1 -> Sum43/1
  Gain3/1 -> Sum5/1
  Sum33/1 -> GainA12/1, Delay23/1
  Sum34/1 -> Sum33/2
  Sum23/1 -> Sum26/1
  Gain23/1 -> Sum34/1
  Delay24/1 -> Gain23/1
  Sum32/1 -> Sum35/1
  GainA12/1 -> Sum35/2
  In1/1 -> Gain33/1
  GainB12/1 -> Sum35/3
  Delay23/1 -> GainB12/1, Gain22/1, Delay24/1
  Gain22/1 -> Sum34/2
  GainA1/1 -> Sum/2
  GainB1/1 -> Sum/3
  GainB4/1 -> Sum9/3
  GainA4/1 -> Sum9/2
  Delay7/1 -> Gain7/1
  Gain7/1 -> Sum11/1
  Sum11/1 -> Sum10/2
  Gain6/1 -> Sum11/2
  Delay8/1 -> GainB4/1, Gain6/1, Delay7/1
  Sum10/1 -> GainA4/1, Delay8/1
  Gain_/1 -> Sum/1
  Gain_1/1 -> Sum49/2
  Sum49/1 -> Sum48/1, Sum2/1, Sum7/1, Sum10/1, Sum12/1, Sum15/1, Sum18/1, Sum21/1, Sum24/1, Sum27/1, Sum30/1, Sum33/1, Sum36/1, Sum39/1, Sum42/1, Sum45/1, Sum62/1, Sum65/1, Sum86/1, Sum89/1, Sum92/1, Sum95/1, Sum83/1, Sum80/1, Sum77/1, Sum74/1, Sum71/1, Sum68/1, Sum59/1, Sum56/1, Sum53/1, Sum50/1, Sum4/1
